simulink model "mpc_motor"  (Simulink 6.0)
settings: Solver=ode45  SolverMode=SingleTasking  StartTime=0.0  StopTime=Tstop  RelTol=1e-3
libraries: mpclib x1, cstblocks x1
settings Model: Creator=jowen  LastModifiedBy=jowen  ExtModeTrigMode=oneshot  ExtModeArmWhenConnect=off
settings DataIOCC: LimitDataPoints=off  SignalLoggingName=sigsOut
settings OptimizationCC: BooleanDataType=off  InlineInvariantSignals=off
settings DebuggingCC: CheckExecutionContextPreStartOutputMsg=on  CheckExecutionContextRuntimeOutputMsg=on  SolverPrmCheckMsg=none  IntegerOverflowMsg=none
settings HardwareCC: TargetUnknown=on
settings GRTTargetCC: ModelReferenceCompliant=off  MatFileLogging=off
settings SFSimCC: SFSimApplyToAllLibs=on  SFSimBuildMode=Incremental

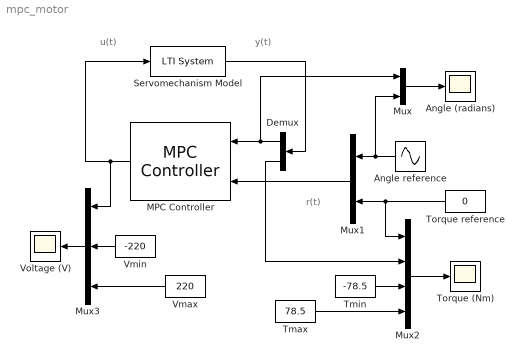
== system mpc_motor ==
  note: u(t)
  note: y(t)
  note: r(t)
  Angle (radians) : Scope
      settings: TimeRange=20  YMin=-4  YMax=4  DataFormat=Structure
  Angle reference : Sin  Orientation=left  Amplitude=pi  Frequency=.4  SampleTime=0
  Demux : Demux  Orientation=left  Outputs=2
  MPC Controller : mpclib/MPC Controller  Orientation=left  mpcobj=ServoMPC  n_mv=0  x0=[]  ref_from_ws=off  ref_signal_name=[]  ref_preview=on  md_from_ws=off  md_signal_name=[]  md_preview=on  from_project=off  md_inport=off  project_file=MPCtask.mat
  Mux : Mux  Inputs=2
  Mux1 : Mux  Orientation=left  Inputs=2
  Mux2 : Mux
  Mux3 : Mux  Orientation=left  Inputs=3
  Servomechanism Model : cstblocks/LTI System  sys=sys  IC=[]
  Tmax : Constant  Value=78.5
  Tmin : Constant  Value=-78.5
  Torque (Nm) : Scope
      settings: TimeRange=20  YMin=-100  YMax=100  DataFormat=Structure
  Torque reference : Constant  Orientation=left  Value=0
  Vmax : Constant  Orientation=left  Value=220
  Vmin : Constant  Orientation=left  Value=-220
  Voltage (V) : Scope
      settings: TimeRange=20  YMin=-250  YMax=250  DataFormat=Structure
  wires:
  MPC Controller/1 -> Servomechanism Model/1, Mux3/1
  Servomechanism Model/1 -> Demux/1
  Mux/1 -> Angle (radians)/1
  Mux2/1 -> Torque (Nm)/1
  Demux/2 -> Mux2/2
  Mux1/1 -> MPC Controller/2
  Angle reference/1 -> Mux1/1, Mux/2
  Demux/1 -> Mux/1, MPC Controller/1
  Mux3/1 -> Voltage (V)/1
  Vmin/1 -> Mux3/2
  Vmax/1 -> Mux3/3
  Tmin/1 -> Mux2/3
  Tmax/1 -> Mux2/4
  Torque reference/1 -> Mux1/2, Mux2/1
